simulink model "simprova"  (R2018b)
settings: Solver=VariableStepAuto  StartTime=0.0  StopTime=10.0  RelTol=1e-3
values from neighbouring files (symbols this model uses):
  c1 = ((a1+a2*c2)*pw_x+a2*s2*pw_y)/(pw_x^2+pw_y^2)    [analitycal_IK_4DoF_v1.m]    (also in initialization_simulazione.m = [25 49.5]; provatraiettoria.m = [25 49.5])
  c2 = (pw_x^2+pw_y^2-a1^2-a2^2)/(2*a1*a2)    [analitycal_IK_4DoF_v1.m]    (also in initialization_simulazione.m = [25 11]; provatraiettoria.m = [25 11])
  r1 = 30    [initialization_simulazione.m]    (also in provatraiettoria.m)
  r2 = 10    [initialization_simulazione.m]    (also in provatraiettoria.m)
settings Model: Creator=camillo  LastModifiedBy=camillo

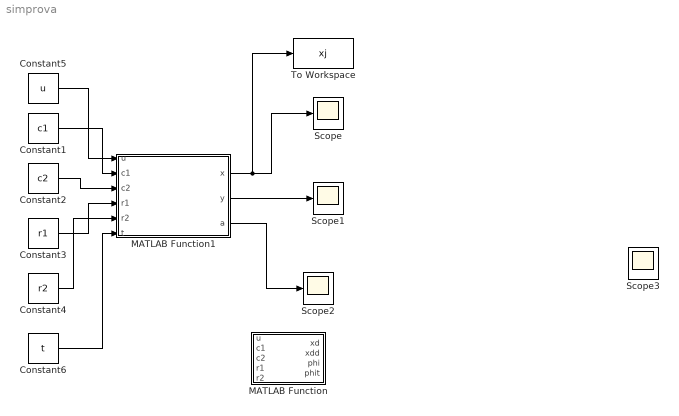
== system simprova ==
  Constant1 : Constant  Value=c1
  Constant2 : Constant  Value=c2
  Constant3 : Constant  Value=r1
  Constant4 : Constant  Value=r2
  Constant5 : Constant  Value=u
  Constant6 : Constant  Value=t
  MATLAB Function : MATLAB Function  TreatAsAtomicUnit=on
  MATLAB Function1 : MATLAB Function  TreatAsAtomicUnit=on
  Scope{,1..3} (4 alike) : Scope
  To Workspace : ToWorkspace  VariableName=xj  SaveFormat=Timeseries  SampleTime=-1
  wires:
  Constant5/1 -> MATLAB Function1/1(u)
  Constant1/1 -> MATLAB Function1/2(c1)
  Constant2/1 -> MATLAB Function1/3(c2)
  Constant3/1 -> MATLAB Function1/4(r1)
  Constant4/1 -> MATLAB Function1/5(r2)
  Constant6/1 -> MATLAB Function1/6(t)
  MATLAB Function1/3(a) -> Scope2/1
  MATLAB Function1/2(y) -> Scope1/1
  MATLAB Function1/1(x) -> To Workspace/1, Scope/1

== matlab function simprova/MATLAB Function1 ==
  data: x output; u input; y output; c1 input; a output; c2 input; r1 input; r2 input; t input
function [x,y,a] = fcn(u,c1,c2,r1,r2,t)
x = zeros(201,1);
y = zeros(201,1);
a = zeros(201,1);
xd = struct;
phi = struct;
for i=1:length(t)
    u(10)=t(i);
    [xd(i).traiettoria,xd(i).derivata,phi(i).orientamento,phi(i).derivata]=...
        planner_TOAD(u,c1,c2,r1,r2);
end

for i=1:length(t)
    x(i)=xd(i).traiettoria(1);
    y(i)=xd(i).traiettoria(2);

    a(i)=phi(i).orientamento;
end
end

== matlab function simprova/MATLAB Function ==
  data: u input; xd output; c1 input; c2 input; r1 input; r2 input; xdd output; phi output; phit output
function [xd, xdd, phi, phit] = fcn(u,c1,c2,r1,r2) %OUT = planner_TOAD(u,c1,c2,r1,r2)%
    xd = zeros(201,2);
    xdd = zeros(201,2);
    phi = zeros(201,1);
    phit = zeros(201,1);
    XYd = zeros(201,2);
    XYddot = zeros(201,2);
    %mi definisco i parametri da utilizzare per la pianificazione della
    %traiettoria e dell'orientamento:
    pf=u(1:2); %punto finale per il primo tratto, coincide con il punto A

    p_i=u(3:4); %punto iniziale per il primo tratto, coincide con il punto B

    ti=u(5); %tempo iniziale

    tf=u(6); %tempo finale per il primo tratto

    tf2=u(7); %tempo finale per il secondo tratto

    t=u(10); %variabile temporale

    phi_i=u(8); %phi iniziale per il primo tratto, ovvero in B

    phi_f=u(9); %phi finale per il primo tratto, ovvero in A

    alfa_2=deg2rad(341); %angolo di rotazione per il primo tratto

    beta=deg2rad(302);

    if t<=tf %se ci troviamo ad un tempo inferiore di tf, dobbiamo pianificare
        %la traiettoria circolare del primo tratto, con raggio 'r1' e centro
        %'c1'
        A_2=[ti^3 ti^2 ti 1;
           tf^3 tf^2 tf 1;
           3*ti^2 2*ti 1 0;
           3*tf^2 2*tf 1 0]; %definisco la matrice dei termini noti temporali, derivante
        %dalle condizioni di definizione della legge oraria 's(t)', essa vale sia
        %per l'orientamento che per la traiettoria
        B_2=[0;r1*alfa_2;0;0]; %vettore dei termini noti per la traiettoria
        a_2=inv(A_2)*B_2; %coefficienti della legge oraria per la traiettoria

        s=a_2(1)*t^3+a_2(2)*t^2+a_2(3)*t+a_2(4); %legge oraria della traiettoria
        sdot=3*a_2(1)*t^2+2*a_2(2)*t+a_2(3); %derivata della legge oraria

        th=deg2rad(-80.5);

        R=[cos(th) -sin(th);
            sin(th) cos(th)];
        %rotazione per la pianificazione di una traiettoria
        %circolare, sappiamo che l'equazione si riferisce ad una terna concentrica
        %a 'c1' e con angolo nullo quando ci troviamo nella situazione s(0)

        B_2phi=[phi_i;phi_f;0;0]; %vettore dei termini noti per l'orientamento
        a_2phi=inv(A_2)*B_2phi; %coefficienti della legge oraria per l'orientamento
        s_phi=a_2phi(1)*t^3+a_2phi(2)*t^2+a_2phi(3)*t+a_2phi(4); %legge oraria orientamento
        sdot_phi=3*a_2phi(1)*t^2+2*a_2phi(2)*t+a_2phi(3); %derivata legge oraria orientamento

        if t<ti %se ci troviamo ad un tempo inferiore a quello iniziale allora ci troviamo nella
            %configurazione iniziale sia per la posizione che per l'orientamento
            XYd=p_i;
            XYddot=[0;0];
            phi_e=phi_i;
            phi_et=0;
        else
            if t<=tf %se ci troviamo tra ti e tf allora definisco la traiettoria
                %circolare e l'orientamento secondo una legge lineare con s_phi:
                XYd=(c1'+R*[r1*cos(s/r1) r1*sin(s/r1)]')'; %è la x desiderata
                XYddot=(R*[-sin(s/r1) cos(s/r1)]')';

                phi_e=phi_i+(s_phi/norm(phi_f-phi_i))*(phi_f-phi_i); %è la phi desiderata
                phi_et=(sdot_phi/norm(phi_f-phi_i))*(phi_f-phi_i);
            %     else %altrimenti rimango alla situazione finale, in realtà si può togliere questa parte
            %     XYd=pf;
            %     XYddot=[0;0];
            %     phi_e=phi_f;
            %     phi_et=0;
            end
        end

    else %se ci troviamo ad un tempo maggiore di tf siamo passati a descrivere
        %la seconda traiettoria:
        A_1=[tf^3 tf^2 tf 1;
           tf2^3 tf2^2 tf2 1;
           3*tf^2 2*tf 1 0;
           3*tf2^2 2*tf2 1 0]; %definisco come prima la matrice A
        B_1=[0;r2*beta;0;0]; %vettore termini noti per la traiettoria 
        a_1=inv(A_1)*B_1; %coefficienti della legge oraria della traiettoria

        s=a_1(1)*t^3+a_1(2)*t^2+a_1(3)*t+a_1(4); %legge oraria traiettoria
        sdot=3*a_1(1)*t^2+2*a_1(2)*t+a_1(3); %derivata legge oraria

        gamma=deg2rad(119);

        R1=[cos(gamma) -sin(gamma);
            sin(gamma) cos(gamma)]; %& pi %matrice di rotazione per rimetterci nelle condizioni
        %per la pianificazione della traiettoria con centro 'c2' e raggio 'r2'

        B_1phi=[phi_i;phi_f;0;0]; %vettore termini noti per l'orientamento
        a_1phi=inv(A_1)*B_1phi; %coefficienti legge oraria orientamento
        s_phi=a_1phi(1)*t^3+a_1phi(2)*t^2+a_1phi(3)*t+a_1phi(4); %legge oraria orientamento
        sdot_phi=3*a_1phi(1)*t^2+2*a_1phi(2)*t+a_1phi(3); %derivata legge oraria orientamento

        if t<=tf2 %se ci troviamo ad un tempo inferiore di tf2 andiamo a pianificare la
                %traiettoria ed orientamento:
            XYd=(c2'+R1*[r2*cos(s/r2) r2*sin(s/r2)]')'; %x desiderata
            XYddot=(R1*[-sin(s/r2) cos(s/r2)]')';

            phi_e=phi_f+(s_phi/norm(phi_i-phi_f))*(phi_i-phi_f); %phi desiderata
            phi_et=(sdot_phi/norm(phi_i-phi_f))*(phi_i-phi_f);

        else %altrimenti rimaniamo alla configurazione da cui siamo partiti ovvero nel punto B
            XYd=p_i;
            XYddot=[0;0];
            phi_e=phi_i;
            phi_et=0;
        end
    end 

    %salvo i dati che voglio in uscita
    xd=XYd;
    xdd=XYddot;
    phi=phi_e;
    phit=phi_et;
    %XYd = [xd, xdd];
    %XYddot = [phi, phit];
    %OUT = [XYd, XYddot];
end
